simulink model "cart_model"  (R2020a)
settings: Solver=VariableStepAuto  StartTime=0.0  StopTime=10.0  RelTol=1e-3
libraries: mpclib x1
settings Model: Creator=abhinav  LastModifiedBy=abhinav

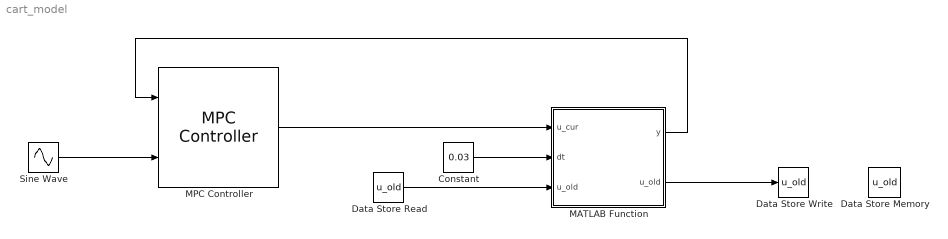
== system cart_model ==
  Constant : Constant  Value=0.03
  Data Store Memory : DataStoreMemory  DataStoreName=u_old  ReadBeforeWriteMsg=warning  WriteAfterWriteMsg=warning  WriteAfterReadMsg=warning  ShowAdditionalParam=off  OutDataTypeStr=double
  Data Store Read : DataStoreRead  DataStoreName=u_old
  Data Store Write : DataStoreWrite  DataStoreName=u_old
  MATLAB Function : MATLAB Function  TreatAsAtomicUnit=on
  MPC Controller : mpclib/MPC Controller  SCDEnableBlockLinearizationSpecification=on  is_multiple=0  enable_value=0  return_u0=off  updateMPCinCallerWorkspace=on  md_inport=off  mv_inport=off  uref_inport=off  return_cost=off  return_mvseq=off  return_qpstatus=off  return_xseq=off  return_state=off  return_ovseq=off  state_inport=off  umin_inport=off  umax_inport=off  ymin_inport=off  ymax_inport=off  cc_inport=off  ywt_inport=off  uwt_inport=off  duwt_inport=off  rhoeps_inport=off  pm_inport=off  MaximumP=10  HorizonChoice=FixedHorizon  n_ts=1  n_p=10  n_mv=1  n_md=1  n_ud=0  n_mo=1  n_uo=0  BlockDataType=double  SampleTimeInherited=off  switch_inport=off
  Sine Wave : Sin  Frequency=30  SampleTime=0
  wires:
  MPC Controller/1 -> MATLAB Function/1(u_cur)
  Constant/1 -> MATLAB Function/2(dt)
  MATLAB Function/1(y) -> MPC Controller/1
  MATLAB Function/2(u_old) -> Data Store Write/1
  Data Store Read/1 -> MATLAB Function/3("u_old ")
  Sine Wave/1 -> MPC Controller/2

== matlab function cart_model/MATLAB Function ==
  data: u_cur input; y output; dt input; u_old output; u_old input
function [y, u_old] = cart(u_cur,dt, u_old)
y = [0, 0];

ux_cur = u_cur(1);
uy_cur = u_cur(2);

ax = (ux_cur - u_old(1))/dt;
ay = (uy_cur - u_old(2))/dt;

u_old(1) = ux_cur;
u_old(2) = uy_cur;

y(1) = ux_cur*dt + 0.5*ax*dt*dt;
y(2) = uy_cur*dt + 0.5*ay*dt*dt;

end
